simulink model "stepResponse"  (Simulink 8.8)
settings: Solver=FixedStepDiscrete  StartTime=0.0  StopTime="Config.SIMULATION_TIME "  FixedStep=Config.Ts  RelTol=1e-3  EnableMultiTasking=on
InitFcn:
  | cd(fileparts(which(bdroot)));
  | init;
StopFcn:
  | cd(fileparts(which(bdroot)));
  | saveData;
values from neighbouring files (symbols this model uses):
  desiredJointPosition = ones(1,ROBOT_DOF)    [init.m]
undefined symbols (not defined in the file or in its folder): Config
libraries: WBToolboxLibrary x6, simulink_extras x2
settings Model: SuppressorTable=22 serialization::archive 11 0 3 0 0 0 11 0  Creator=daniele  LastModifiedBy=giulio
settings DataIOCC: SignalLoggingSaveFormat=Dataset
settings OptimizationCC: ExpressionDepthLimit=2147483647
settings DebuggingCC: SolverPrmCheckMsg=warning  AllowSymbolicDim=off
settings SFSimCC: SimParseCustomCode=off

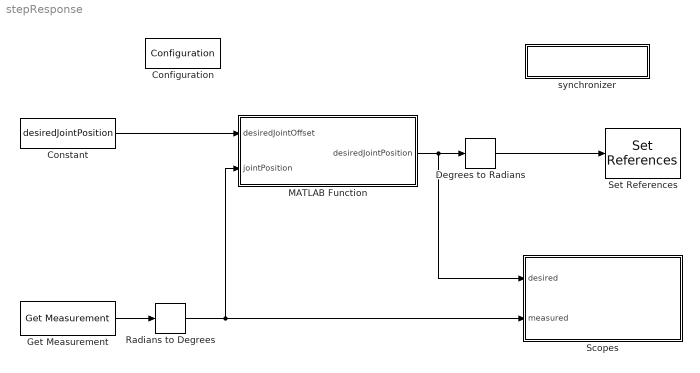
== system stepResponse ==
  Configuration : WBToolboxLibrary/Utilities/Configuration  ConfigSource=Workspace  ConfigObject='WBTConfigRobot'
  Constant : Constant  Value=desiredJointPosition
  Degrees to Radians : simulink_extras/Transformations/Degrees to Radians
  Get Measurement : WBToolboxLibrary/wholeBodyStates/Get Measurement  measuredType=Joints Position
  MATLAB Function : MATLAB Function  TreatAsAtomicUnit=on
  Radians to Degrees : simulink_extras/Transformations/Radians to Degrees
  Scopes : Subsystem
  Set References : WBToolboxLibrary/wholeBodyActuators/Set References  controlType=Position Direct  refSpeed=10*(pi/180)  refAcceleration=1000000*(pi/180)
  synchronizer : Subsystem
      mask Display: disp('SYNCHRONIZER')
  wires:
  Get Measurement/1 -> Radians to Degrees/1
  Degrees to Radians/1 -> Set References/1
  Radians to Degrees/1 -> MATLAB Function/2(jointPosition), Scopes/2("measured ")
  Constant/1 -> MATLAB Function/1(desiredJointOffset)
  MATLAB Function/1(desiredJointPosition) -> Scopes/1(desired), Degrees to Radians/1

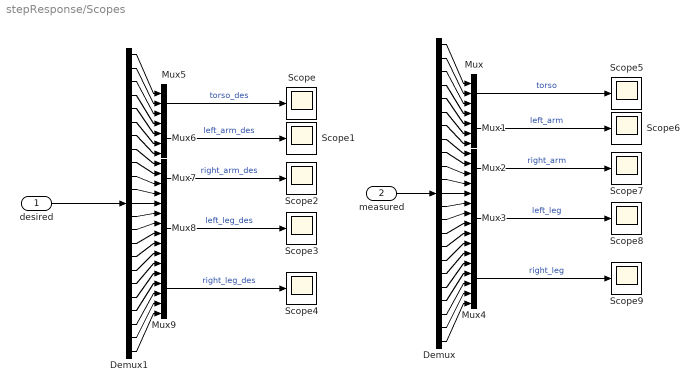
== system stepResponse/Scopes ==
  desired : Inport
  "measured " : Inport  Port=2
  Demux : Demux  Outputs=23
  Demux1 : Demux  Outputs=23
  Mux : Mux  Inputs=3
  Mux{1..2,6..7} (4 alike) : Mux
  Mux{3..4,8..9} (4 alike) : Mux  Inputs=6
  Mux5 : Mux  Inputs=3
  Scope{,1..9} (10 alike) : Scope
  wires:
  Demux/22 -> Mux4/5
  Demux/3 -> Mux/3
  Demux1/15 -> Mux8/4
  Demux/17 -> Mux3/6
  Demux/19 -> Mux4/2
  Demux/21 -> Mux4/4
  Demux1/23 -> Mux9/6
  Demux/8 -> Mux2/1
  Demux/9 -> Mux2/2
  Mux6/1 -> Scope1/1  "left_arm_des"
  Demux/10 -> Mux2/3
  Demux/11 -> Mux2/4
  Demux1/17 -> Mux8/6
  Demux/2 -> Mux/2
  Demux/20 -> Mux4/3
  Demux/7 -> Mux1/4
  Demux1/13 -> Mux8/2
  Demux1/11 -> Mux7/4
  Demux1/20 -> Mux9/3
  Mux5/1 -> Scope/1  "torso_des"
  Demux1/4 -> Mux6/1
  Demux/18 -> Mux4/1
  Demux1/12 -> Mux8/1
  Demux1/3 -> Mux5/3
  Demux1/1 -> Mux5/1
  Demux1/19 -> Mux9/2
  "measured "/1 -> Demux/1
  Demux1/2 -> Mux5/2
  Demux1/18 -> Mux9/1
  Demux1/16 -> Mux8/5
  Demux1/8 -> Mux7/1
  Demux1/9 -> Mux7/2
  Demux/23 -> Mux4/6
  Demux/4 -> Mux1/1
  Mux9/1 -> Scope4/1  "right_leg_des"
  Demux1/5 -> Mux6/2
  Demux1/21 -> Mux9/4
  Demux1/10 -> Mux7/3
  Demux1/7 -> Mux6/4
  Demux1/14 -> Mux8/3
  Demux1/6 -> Mux6/3
  Demux/1 -> Mux/1
  Demux1/22 -> Mux9/5
  Demux/16 -> Mux3/5
  Demux/15 -> Mux3/4
  Demux/6 -> Mux1/3
  Demux/5 -> Mux1/2
  Demux/14 -> Mux3/3
  Demux/12 -> Mux3/1
  Demux/13 -> Mux3/2
  desired/1 -> Demux1/1
  Mux8/1 -> Scope3/1  "left_leg_des"
  Mux7/1 -> Scope2/1  "right_arm_des"
  Mux1/1 -> Scope6/1  "left_arm"
  Mux/1 -> Scope5/1  "torso"
  Mux4/1 -> Scope9/1  "right_leg"
  Mux3/1 -> Scope8/1  "left_leg"
  Mux2/1 -> Scope7/1  "right_arm"

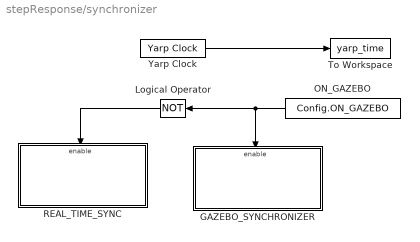
== system stepResponse/synchronizer ==
  GAZEBO_SYNCHRONIZER : Subsystem
  Logical Operator : Logic  Operator=NOT  AllPortsSameDT=off  OutDataTypeStr=boolean
  "ON_GAZEBO " : Constant  Value=Config.ON_GAZEBO
  REAL_TIME_SYNC : Subsystem
  To Workspace : ToWorkspace  VariableName=yarp_time  SaveFormat=Structure With Time  SampleTime=-1
  Yarp Clock : WBToolboxLibrary/Utilities/Yarp Clock
  wires:
  Logical Operator/1 -> REAL_TIME_SYNC/Enable
  "ON_GAZEBO "/1 -> GAZEBO_SYNCHRONIZER/Enable, Logical Operator/1
  Yarp Clock/1 -> To Workspace/1

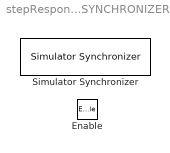
== system stepResponse/synchronizer/GAZEBO_SYNCHRONIZER ==
  Enable : EnablePort
  Simulator Synchronizer : WBToolboxLibrary/Utilities/Simulator Synchronizer  period=Config.Ts  serverPortName='/clock/rpc'  clientPortName='/WBT_synchronizer/rpc:o'

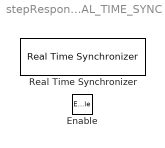
== system stepResponse/synchronizer/REAL_TIME_SYNC ==
  Enable : EnablePort
  Real Time Synchronizer : WBToolboxLibrary/Utilities/Real Time Synchronizer  period=Config.Ts

== matlab function MATLAB Function ==
  data: desiredJointOffset input double; desiredJointPosition output double; jointPosition input double
function desiredJointPosition = setJoint(desiredJointOffset, jointPosition)
persistent initialJointPosition;
if isempty(initialJointPosition)
 initialJointPosition = jointPosition;
end

desiredJointPosition = desiredJointOffset + initialJointPosition;

end
